simulink subsystem "milestone2_maze"  (R2025b)
settings: Solver=VariableStepAuto  StartTime=0.0  StopTime=10.0  RelTol=1e-3
InitFcn:
  | simstruct_init(0);
StartFcn:
  | proj_root = fileparts(fileparts(fileparts(which('launch_virtual_testbed.m')))); fid = fopen(fullfile(proj_root, 'firmware', 'build', 'matlab_callbacks.log'), 'a'); if fid ~= -1, fprintf(fid, '%s: StartFcn triggered\n', datestr(now)); fclose(fid); end; run(which('launch_virtual_testbed.m'));
StopFcn:
  | proj_root = fileparts(fileparts(fileparts(which('launch_virtual_testbed.m')))); fid = fopen(fullfile(proj_root, 'firmware', 'build', 'matlab_callbacks.log'), 'a'); if fid ~= -1, fprintf(fid, '%s: StopFcn triggered\n', datestr(now)); fclose(fid); end; clear mex; clear functions; if ~ispc, [~, ~] = system('/usr/bin/pkill -f ''[p]hysics_sim.py'' '); else, [~, ~] = system('powershell -Command \"Get-CimInstance Win32_Process -Filter \\\"CommandLine like ''%physics_sim.py%''\\\" | Invoke-CimMethod -MethodName Terminate\" >nul 2>&1'); end
settings Model: Creator=JesseJabezArendse  LastModifiedBy=nicolls
settings RTWCC: GenCodeOnly=on  PostCodeGenCommand=flash_micromouse(buildInfo)

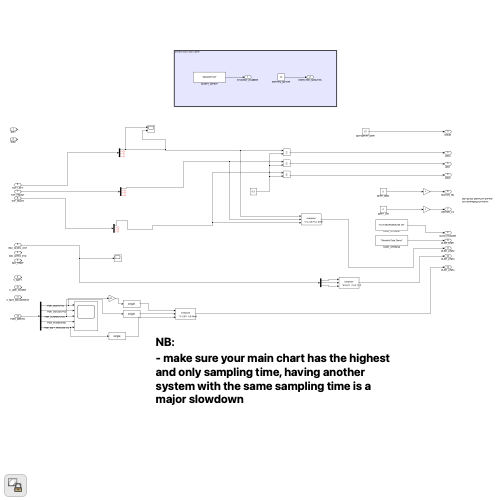
[thumbnail: Simulink's stored preview of the top-level diagram]
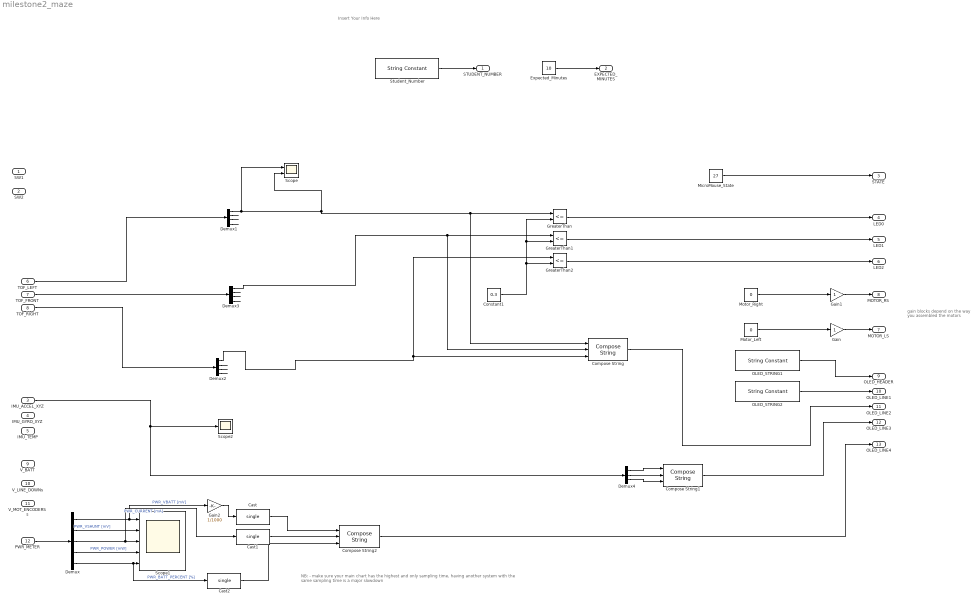
== system milestone2_maze ==
  note: NB:
      |
      | - make sure your main chart has the highest and only sampling time, having another system with the same sampling time is a major slowdown
  note: gain blocks depend on the way
      | you assembled the motors
  note: Insert Your Info Here
  SW1 : Inport
  SW2 : Inport  Port=2
  IMU_ACCEL_XYZ : Inport  Port=3
  IMU_GYRO_XYZ : Inport  Port=4
  IMU_TEMP : Inport  Port=5
  TOF_LEFT : Inport  Port=6
  TOF_FRONT : Inport  Port=7
  TOF_RIGHT : Inport  Port=8
  V_BATT : Inport  Port=9
  V_LINE_DOWNs : Inport  Port=10
  V_MOT_ENCODERSs : Inport  Port=11
  PWR_METER : Inport  Port=12
  Cast : DataTypeConversion  OutDataTypeStr=single  SaturateOnIntegerOverflow=off  RndMeth=Floor
  Cast1 : DataTypeConversion  OutDataTypeStr=single  SaturateOnIntegerOverflow=off  RndMeth=Floor
  Cast2 : DataTypeConversion  OutDataTypeStr=single  SaturateOnIntegerOverflow=off  RndMeth=Floor
  Compose String : ComposeString  Format="\"L%1.2f F%1.2f R%1.2f\""
  Compose String1 : ComposeString  Format="\"X%2.1f  Y%2.1f  Z%2.1f\""
  Compose String2 : ComposeString  Format="\"%1.2fV  %3.0fmA  %2.0f%%\""
  Constant1 : Constant  Value=0.3  SampleTime=-1
  Demux : Demux  Outputs=5
  Demux1 : Demux
  Demux2 : Demux
  Demux3 : Demux
  Demux4 : Demux  Outputs=3
  Expected_Minutes : Constant  Value=10  OutDataTypeStr=uint8
  Gain : Gain  OutDataTypeStr=Inherit: Same as input
  Gain1 : Gain  OutDataTypeStr=Inherit: Same as input
  Gain2 : Gain  Gain=1/1000
  GreaterThan : RelationalOperator  Operator=<=  OutDataTypeStr=boolean  RndMeth=Simplest  InputSameDT=off
  GreaterThan1 : RelationalOperator  Operator=<=  OutDataTypeStr=boolean  RndMeth=Simplest  InputSameDT=off
  GreaterThan2 : RelationalOperator  Operator=<=  OutDataTypeStr=boolean  RndMeth=Simplest  InputSameDT=off
  MicroMouse_State : Constant  Value=27
  Motor_Left : Constant  Value=0
  Motor_Right : Constant  Value=0
  OLED_STRING1 : StringConstant  String="\"UCT MICROMOUSE '25\""
  OLED_STRING2 : StringConstant  String="\"Simulink Data Demo\""
  Scope : Scope  NumInputPorts=2
      settings: ActiveDisplayYMinimum=0.22759  ActiveDisplayYMaximum=0.52326
  Scope1 : Scope  NumInputPorts=5
      settings: ActiveDisplayYMinimum=-437.5  ActiveDisplayYMaximum=3937.5  DataLoggingVariableName=ScopeData2
  Scope2 : Scope
  Student_Number : StringConstant  String="\"ABCDEF123\""
  STUDENT_NUMBER : Outport
  EXPECTED_MINUTES : Outport  Port=2
  STATE : Outport  Port=3
  LED0 : Outport  Port=4
  LED1 : Outport  Port=5
  LED2 : Outport  Port=6
  MOTOR_LS : Outport  Port=7
  MOTOR_RS : Outport  Port=8
  OLED_HEADER : Outport  Port=9
  OLED_LINE1 : Outport  Port=10
  OLED_LINE2 : Outport  Port=11
  OLED_LINE3 : Outport  Port=12
  OLED_LINE4 : Outport  Port=13
  wires:
  TOF_FRONT/1 -> Demux3/1
  OLED_STRING2/1 -> OLED_LINE1/1
  Demux2/3 -> ?
  Demux2/2 -> ?
  Demux2/4 -> ?
  Compose String1/1 -> OLED_LINE3/1
  Demux3/1 -> Compose String/2, GreaterThan1/1
  GreaterThan1/1 -> LED1/1
  Demux3/3 -> ?
  TOF_RIGHT/1 -> Demux2/1
  Demux3/4 -> ?
  Demux3/2 -> ?
  Demux1/2 -> ?
  OLED_STRING1/1 -> OLED_HEADER/1
  Compose String/1 -> OLED_LINE2/1
  Constant1/1 -> GreaterThan2/2, GreaterThan1/2, GreaterThan/2
  Demux1/4 -> ?
  GreaterThan2/1 -> LED2/1
  TOF_LEFT/1 -> Demux1/1
  GreaterThan/1 -> LED0/1
  Demux1/3 -> ?
  PWR_METER/1 -> Demux/1
  Demux/1 -> Scope1/1, Gain2/1  "PWR_VBATT [mV]"
  Demux/2 -> Scope1/2  "PWR_VSHUNT [mV]"
  Demux/3 -> Scope1/3, Cast1/1  "PWR_CURRENT [mA]"
  Demux/4 -> Scope1/4  "PWR_POWER [mW]"
  Demux/5 -> Scope1/5, Cast2/1  "PWR_BATT_PERCENT [%]"
  IMU_ACCEL_XYZ/1 -> Demux4/1, Scope2/1
  Demux4/1 -> Compose String1/1
  Demux4/2 -> Compose String1/2
  Demux4/3 -> Compose String1/3
  Compose String2/1 -> OLED_LINE4/1
  Gain2/1 -> Cast/1
  Cast/1 -> Compose String2/1
  Cast1/1 -> Compose String2/2
  Cast2/1 -> Compose String2/3
  Demux2/1 -> Compose String/3, GreaterThan2/1
  Demux1/1 -> Scope/1, Scope/2, Compose String/1, GreaterThan/1
  MicroMouse_State/1 -> STATE/1
  Motor_Right/1 -> Gain1/1
  Motor_Left/1 -> Gain/1
  Gain/1 -> MOTOR_LS/1
  Gain1/1 -> MOTOR_RS/1
  Student_Number/1 -> STUDENT_NUMBER/1
  Expected_Minutes/1 -> EXPECTED_MINUTES/1
